simulink model "flug2d2"  (Simulink 7.0)
settings: Solver=ode45  StartTime=0.0  StopTime=700  RelTol=1e-3
libraries: kalmanlib x2, simulink x2
settings Model: Creator=peter  LastModifiedBy=peter  ExtModeAutoUpdateStatusClock=off

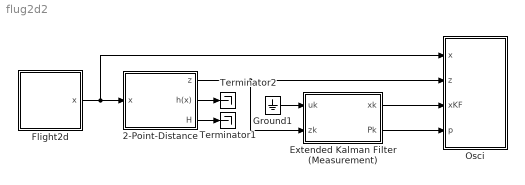
== system flug2d2 ==
  2-Point-Distance : Subsystem  mask(twoPointDistance){P1=[1000;4000], P2=[3000;0], R=diag([1 1 0.003 0.003]), dt=1, seed=[1 2 3 4]'}
      mask prompts: P1 "1. Bezugspunkt"; P2 "2. Bezugspunkt"; R "variance of  measurement noise R"; dt "sample time"; seed "initial seed"
      mask help:
      | Measurement z = h(x) given by the distance to two fixed points P1, P2.
      | Assumes input vector of the form (x, y, vx, vy, ax, ay).
      |
      | returns h(x) and the Jacobi Matrix H
  Extended Kalman Filter (Measurement) : Subsystem  mask(Kalman Filter){A=kron([1, 1, 0.5; 0, 1, 1;  0, 0, 1], [1, 0; 0, 1]), B=0, Q=kron([0.050,0.125,0.167; 0.125,0.333,0.500; 0.167,0.500,1.000],[1, 0; 0, 1])*0.001, R=[1 0 0 0; 0 1 0 0; 0 0 0.003 0; 0 0 0 0.003], x0=[50 4001 0 0 0 0]', P0=diag([1 1 1 1 1 1])*1e-2}
      mask prompts: A "Übertragungsmatrix A"; B "Kontrollmatrix B"; Q "Varianz der x-Störung Q"; R "Varianz der y-Störung R"; x0 "geschätzter Anfangsvektor x0"; P0 "geschätzte x-Anfangsvarianz P"
      mask Display:
      | disp('EKF (M)')
      | port_label('input', 1, 'u')
      | port_label('input', 2, 'z')
      | port_label('output', 1, 'x')
      | port_label('output', 2, 'P')
  Flight2d : Subsystem  mask(Flight2D){xS=[50;4000], xL=[4500;50], tS=50, tL=70, v0=10, q=0.001, dt=1, seed=17, s=0, tF=0, e=0}
      mask prompts: xS "start point"; xL "landing point"; tS "duration of start"; tL "duration of landing"; v0 "cruise velocity"; q "variance of acceleration"; dt "sample time"; seed "initial seed"; s "total distance"; tF "cruise time"; e "cruise vector"
      mask init:
      | s = norm(xL - xS);
      | tF = (s - v0/2*(tS + tL))/v0;
      | e = (xL - xS)/s;
      mask Display:
      | plot([0.1 0.8], [0.1 0.9])
      | patch(0.1 + 0.05*cos(0:0.2:2*pi), 0.1 + 0.05*sin(0:0.2:2*pi), [1 0 0])
      | patch(0.8 + 0.05*cos(0:0.2:2*pi), 0.9 + 0.05*sin(0:0.2:2*pi), [1 0 0])
      | port_label('output', 1, 'x')
  Ground1 : Ground
  Osci : Subsystem
      settings: OpenFcn=open_system(find_system(gcbh, 'Name', 'Scope'), 'force')
  Terminator1 : Terminator
  Terminator2 : Terminator
  wires:
  Flight2d/1(x) -> 2-Point-Distance/1(x), Osci/1(x)
  Ground1/1 -> Extended Kalman Filter (Measurement)/1(uk)
  2-Point-Distance/1(z) -> Extended Kalman Filter (Measurement)/2(zk), Osci/2(z)
  Extended Kalman Filter (Measurement)/1(xk) -> Osci/3(xKF)
  Extended Kalman Filter (Measurement)/2(Pk) -> Osci/4(p)
  2-Point-Distance/2(h(x)) -> Terminator2/1
  2-Point-Distance/3(H) -> Terminator1/1

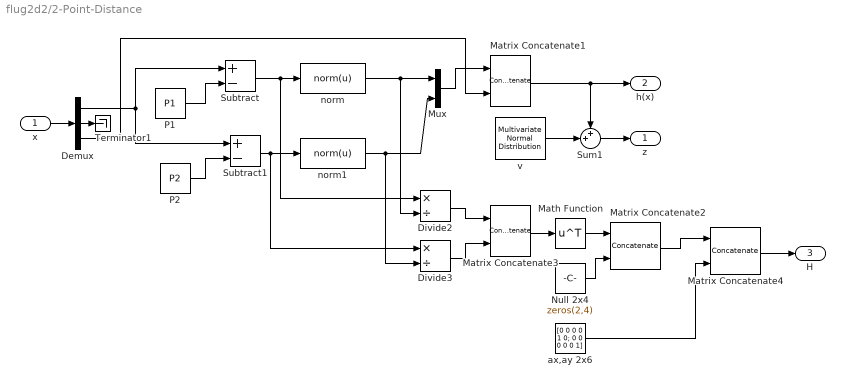
== system flug2d2/2-Point-Distance ==
  x : Inport  OutDataType=sfix(16)  OutScaling=2^0
  Demux : Demux  Outputs=3
  Divide2 : Product  Inputs=*/  OutDataType=sfix(16)  OutScaling=2^-10
  Divide3 : Product  Inputs=*/  OutDataType=sfix(16)  OutScaling=2^-10
  Math Function : Math  Operator=transpose  OutDataType=sfix(16)  OutScaling=2^0  SaturateOnIntegerOverflow=on
  Matrix Concatenate1 : Concatenate  Mode=Multidimensional array
  Matrix Concatenate2 : Concatenate  Mode=Multidimensional array  ConcatenateDimension=2
  Matrix Concatenate3 : Concatenate  Mode=Multidimensional array  ConcatenateDimension=2
  Matrix Concatenate4 : Concatenate  Mode=Multidimensional array
  Mux : Mux  Inputs=2
  Null 2x4 : Constant  Value=zeros(2,4)  VectorParams1D=off  OutDataType=sfix(16)  OutScaling=2^0
  P1 : Constant  Value=P1  VectorParams1D=off  OutDataType=sfix(16)  OutScaling=2^0
  P2 : Constant  Value=P2  VectorParams1D=off  OutDataType=sfix(16)  OutScaling=2^0
  Subtract : Sum  Inputs=+-  OutDataType=sfix(16)  OutScaling=2^-10
  Subtract1 : Sum  Inputs=+-  OutDataType=sfix(16)  OutScaling=2^-10
  Sum1 : Sum  Inputs=++|  OutDataType=sfix(16)  OutScaling=2^0
  Terminator1 : Terminator
  ax,ay 2x6 : Constant  Value=[0 0 0 0 1 0; 0 0 0 0 0 1]  VectorParams1D=off  OutDataType=sfix(16)  OutScaling=2^0
  norm : MATLABFcn  MATLABFcn=norm(u)  OutputDimensions=1
  norm1 : MATLABFcn  MATLABFcn=norm(u)  OutputDimensions=1
  v : kalmanlib/auxiliary/Multivariate Normal  Distribution  SystemSampleTime=-1  m=0  P=R  seed=seed  tS=dt  C=0
  z : Outport  OutDataType=sfix(16)  OutScaling=2^0
  h(x) : Outport  Port=2  OutDataType=sfix(16)  OutScaling=2^0
  H : Outport  Port=3  OutDataType=sfix(16)  OutScaling=2^0
  wires:
  Matrix Concatenate3/1 -> Math Function/1
  Null 2x4/1 -> Matrix Concatenate2/2
  Divide3/1 -> Matrix Concatenate3/2
  Divide2/1 -> Matrix Concatenate3/1
  norm1/1 -> Divide3/2, Mux/2
  norm/1 -> Divide2/2, Mux/1
  Subtract1/1 -> Divide3/1, norm1/1
  Subtract/1 -> Divide2/1, norm/1
  P2/1 -> Subtract1/2
  P1/1 -> Subtract/2
  Demux/1 -> Subtract/1, Subtract1/1
  x/1 -> Demux/1
  Sum1/1 -> z/1
  v/1 -> Sum1/2
  Math Function/1 -> Matrix Concatenate2/1
  Demux/2 -> Terminator1/1
  Mux/1 -> Matrix Concatenate1/1
  Demux/3 -> Matrix Concatenate1/2
  Matrix Concatenate1/1 -> Sum1/1, h(x)/1
  Matrix Concatenate2/1 -> Matrix Concatenate4/1
  ax,ay 2x6/1 -> Matrix Concatenate4/2
  Matrix Concatenate4/1 -> H/1

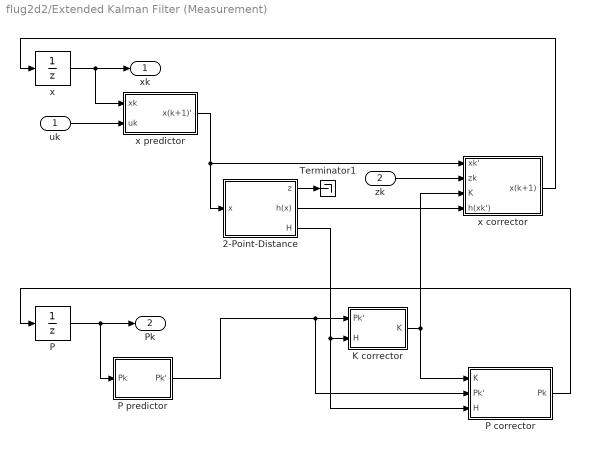
== system flug2d2/Extended Kalman Filter (Measurement) ==
  uk : Inport  OutDataType=sfix(16)  OutScaling=2^0
  zk : Inport  Port=2  OutDataType=sfix(16)  OutScaling=2^0
  2-Point-Distance : Subsystem  mask(twoPointDistance){P1=[1000;4000], P2=[3000;0], R=R, dt=1, seed=[1 2 3 4]'}
      mask prompts: P1 "1. Bezugspunkt"; P2 "2. Bezugspunkt"; R "variance of  measurement noise R"; dt "sample time"; seed "initial seed"
      mask help:
      | Measurement z = h(x) given by the distance to two fixed points P1, P2.
      | Assumes input vector of the form (x, y, vx, vy, ax, ay).
      |
      | returns h(x) and the Jacobi Matrix H
  K corrector : Subsystem
  P : UnitDelay  X0=P0  SampleTime=-1
  P corrector : Subsystem
  P predictor : Subsystem
  Terminator1 : Terminator
  x : UnitDelay  X0=x0  SampleTime=-1
  x corrector : Subsystem
  x predictor : Subsystem
  xk : Outport  OutDataType=sfix(16)  OutScaling=2^0
  Pk : Outport  Port=2  OutDataType=sfix(16)  OutScaling=2^0
  wires:
  2-Point-Distance/3(H) -> P corrector/3(H), K corrector/2(H)
  2-Point-Distance/2(h(x)) -> x corrector/4(h(xk'))
  x corrector/1(x(k+1)) -> x/1
  x/1 -> x predictor/1(xk), xk/1
  P corrector/1(Pk) -> P/1
  K corrector/1(K) -> P corrector/1(K), x corrector/3(K)
  P predictor/1(Pk') -> K corrector/1(Pk'), P corrector/2(Pk')
  P/1 -> Pk/1, P predictor/1(Pk)
  x predictor/1(x(k+1)') -> x corrector/1(xk'), 2-Point-Distance/1(x)
  zk/1 -> x corrector/2(zk)
  uk/1 -> x predictor/2(uk)
  2-Point-Distance/1(z) -> Terminator1/1

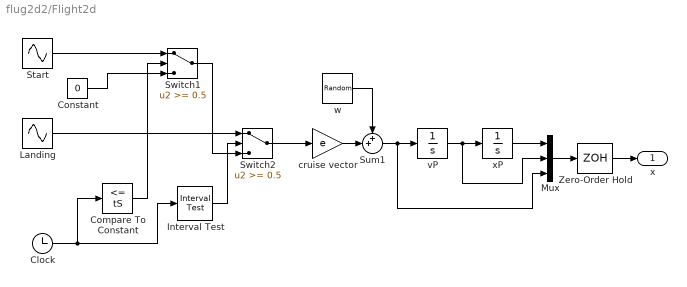
== system flug2d2/Flight2d ==
  Clock : Clock
      settings: Decimation=10
  Compare To Constant : simulink/Logic and Bit Operations/Compare To Constant  SystemSampleTime=-1  relop=<=  const=tS  LogicOutDataTypeMode=boolean  ZeroCross=off
  Constant : Constant  Value=0  OutDataType=sfix(16)  OutScaling=2^0
  Interval Test : simulink/Logic and Bit Operations/Interval Test  SystemSampleTime=-1  IntervalClosedRight=on  uplimit=tS+tF+tL  IntervalClosedLeft=on  lowlimit=tS+tF  LogicOutDataTypeMode=boolean
  Landing : Sin  Amplitude=-v0*pi/(2*tL)  Frequency=pi/tL  Phase=-pi*(tS+tF)/tL  SampleTime=0
  Mux : Mux  Inputs=3
  Start : Sin  Amplitude=v0*pi/(2*tS)  Frequency=pi/tS  SampleTime=0
  Sum1 : Sum  Inputs=++|  OutDataType=sfix(16)  OutScaling=2^0
  Switch1 : Switch  Threshold=0.5
  Switch2 : Switch  Threshold=0.5
  Zero-Order Hold : ZeroOrderHold  SampleTime=dt
  cruise vector : Gain  Gain=e  ParameterDataType=sfix(16)  ParameterScaling=2^0  OutDataType=sfix(16)  OutScaling=2^0
  vP : Integrator  InitialCondition=[0;0]
  w : RandomNumber  Variance=q  Seed=[seed; seed+1]  SampleTime=dt  VectorParams1D=off
  xP : Integrator  InitialCondition=xS
  x : Outport  OutDataType=sfix(16)  OutScaling=2^0
  wires:
  Start/1 -> Switch1/1
  Constant/1 -> Switch1/3
  Compare To Constant/1 -> Switch1/2
  Clock/1 -> Compare To Constant/1, Interval Test/1
  Interval Test/1 -> Switch2/2
  Switch1/1 -> Switch2/3
  Landing/1 -> Switch2/1
  vP/1 -> xP/1, Mux/2
  xP/1 -> Mux/1
  Mux/1 -> Zero-Order Hold/1
  Switch2/1 -> cruise vector/1
  Sum1/1 -> vP/1, Mux/3
  w/1 -> Sum1/1
  Zero-Order Hold/1 -> x/1
  cruise vector/1 -> Sum1/2

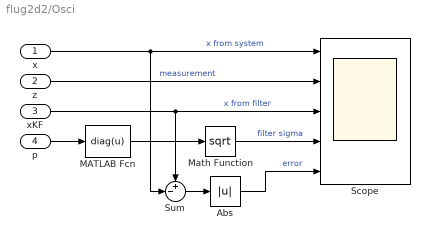
== system flug2d2/Osci ==
  x : Inport  OutDataType=sfix(16)  OutScaling=2^0
  z : Inport  Port=2  OutDataType=sfix(16)  OutScaling=2^0
  xKF : Inport  Port=3  OutDataType=sfix(16)  OutScaling=2^0
  p : Inport  Port=4  OutDataType=sfix(16)  OutScaling=2^0
  Abs : Abs
  MATLAB Fcn : MATLABFcn  MATLABFcn=diag(u)
  Math Function : Math  Operator=sqrt  OutDataType=sfix(16)  OutScaling=2^0  SaturateOnIntegerOverflow=on
  Scope : Scope  NumInputPorts=5
      settings: TimeRange=700  YMin=-1000~-1000~-1000~0~0  YMax=5000~6000~5000~10~30
  Sum : Sum  Inputs=+-|  OutDataType=sfix(16)  OutScaling=2^0
  wires:
  p/1 -> MATLAB Fcn/1
  xKF/1 -> Sum/1, Scope/3  "x from filter"
  z/1 -> Scope/2  "measurement"
  x/1 -> Sum/2, Scope/1  "x from system"
  Abs/1 -> Scope/5  "error"
  Sum/1 -> Abs/1
  Math Function/1 -> Scope/4  "filter sigma"
  MATLAB Fcn/1 -> Math Function/1

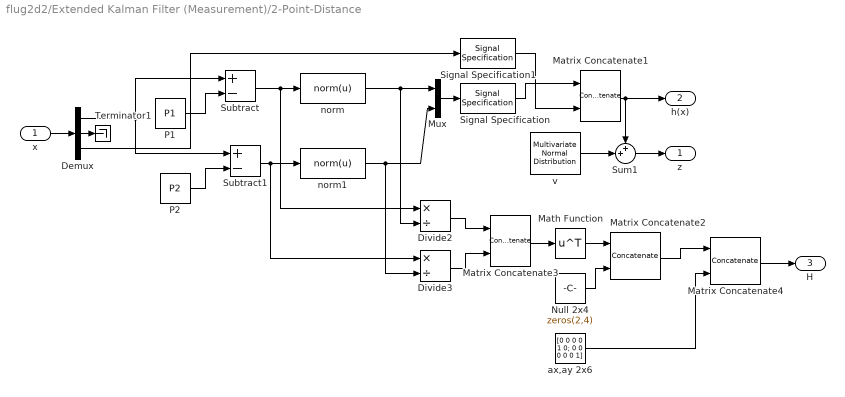
== system flug2d2/Extended Kalman Filter (Measurement)/2-Point-Distance ==
  x : Inport  OutDataType=sfix(16)  OutScaling=2^0
  Demux : Demux  Outputs=3
  Divide2 : Product  Inputs=*/  OutDataType=sfix(16)  OutScaling=2^-10
  Divide3 : Product  Inputs=*/  OutDataType=sfix(16)  OutScaling=2^-10
  Math Function : Math  Operator=transpose  OutDataType=sfix(16)  OutScaling=2^0  SaturateOnIntegerOverflow=on
  Matrix Concatenate1 : Concatenate  Mode=Multidimensional array
  Matrix Concatenate2 : Concatenate  Mode=Multidimensional array  ConcatenateDimension=2
  Matrix Concatenate3 : Concatenate  Mode=Multidimensional array  ConcatenateDimension=2
  Matrix Concatenate4 : Concatenate  Mode=Multidimensional array
  Mux : Mux  Inputs=2
  Null 2x4 : Constant  Value=zeros(2,4)  VectorParams1D=off  OutDataType=sfix(16)  OutScaling=2^0
  P1 : Constant  Value=P1  VectorParams1D=off  OutDataType=sfix(16)  OutScaling=2^0
  P2 : Constant  Value=P2  VectorParams1D=off  OutDataType=sfix(16)  OutScaling=2^0
  Signal Specification : SignalSpecification  Dimensions=[2 1]  OutDataType=sfix(16)  OutScaling=2^0
  Signal Specification1 : SignalSpecification  Dimensions=[2 1]  OutDataType=sfix(16)  OutScaling=2^0
  Subtract : Sum  Inputs=+-  OutDataType=sfix(16)  OutScaling=2^-10
  Subtract1 : Sum  Inputs=+-  OutDataType=sfix(16)  OutScaling=2^-10
  Sum1 : Sum  Inputs=++|  OutDataType=sfix(16)  OutScaling=2^0
  Terminator1 : Terminator
  ax,ay 2x6 : Constant  Value=[0 0 0 0 1 0; 0 0 0 0 0 1]  VectorParams1D=off  OutDataType=sfix(16)  OutScaling=2^0
  norm : MATLABFcn  MATLABFcn=norm(u)  OutputDimensions=1
  norm1 : MATLABFcn  MATLABFcn=norm(u)  OutputDimensions=1
  v : kalmanlib/auxiliary/Multivariate Normal  Distribution  SystemSampleTime=-1  m=0  P=R  seed=seed  tS=dt  C=0
  z : Outport  OutDataType=sfix(16)  OutScaling=2^0
  h(x) : Outport  Port=2  OutDataType=sfix(16)  OutScaling=2^0
  H : Outport  Port=3  OutDataType=sfix(16)  OutScaling=2^0
  wires:
  Signal Specification1/1 -> Matrix Concatenate1/2
  Signal Specification/1 -> Matrix Concatenate1/1
  Matrix Concatenate4/1 -> H/1
  ax,ay 2x6/1 -> Matrix Concatenate4/2
  Matrix Concatenate2/1 -> Matrix Concatenate4/1
  Matrix Concatenate1/1 -> h(x)/1, Sum1/1
  Demux/3 -> Signal Specification1/1
  Mux/1 -> Signal Specification/1
  Demux/2 -> Terminator1/1
  Math Function/1 -> Matrix Concatenate2/1
  v/1 -> Sum1/2
  Sum1/1 -> z/1
  x/1 -> Demux/1
  Demux/1 -> Subtract1/1, Subtract/1
  P1/1 -> Subtract/2
  P2/1 -> Subtract1/2
  Subtract/1 -> norm/1, Divide2/1
  Subtract1/1 -> norm1/1, Divide3/1
  norm/1 -> Mux/1, Divide2/2
  norm1/1 -> Mux/2, Divide3/2
  Divide2/1 -> Matrix Concatenate3/1
  Divide3/1 -> Matrix Concatenate3/2
  Null 2x4/1 -> Matrix Concatenate2/2
  Matrix Concatenate3/1 -> Math Function/1

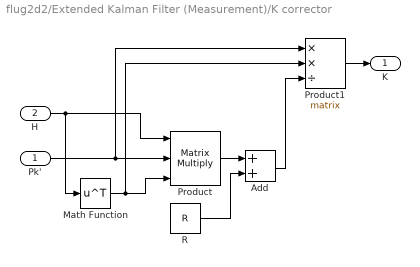
== system flug2d2/Extended Kalman Filter (Measurement)/K corrector ==
  Pk' : Inport  OutDataType=sfix(16)  OutScaling=2^0
  H : Inport  Port=2  OutDataType=sfix(16)  OutScaling=2^0
  Add : Sum  OutDataType=sfix(16)  OutScaling=2^-10
  Math Function : Math  Operator=transpose  OutDataType=sfix(16)  OutScaling=2^0  SaturateOnIntegerOverflow=on
  Product : Product  Inputs=3  Multiplication=Matrix(*)  OutDataType=sfix(16)  OutScaling=2^0  RndMeth=Zero
  Product1 : Product  Inputs=**/  Multiplication=Matrix(*)  OutDataType=sfix(16)  OutScaling=2^0  RndMeth=Zero
  R : Constant  Value=R  OutDataType=sfix(16)  OutScaling=2^0
  K : Outport  OutDataType=sfix(16)  OutScaling=2^0
  wires:
  Add/1 -> Product1/3
  Product1/1 -> K/1
  H/1 -> Math Function/1, Product/1
  Pk'/1 -> Product1/1, Product/2
  Math Function/1 -> Product1/2, Product/3
  Product/1 -> Add/1
  R/1 -> Add/2

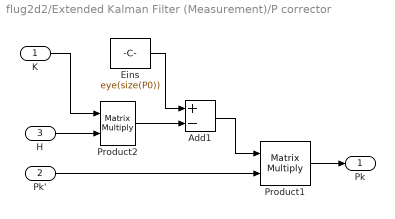
== system flug2d2/Extended Kalman Filter (Measurement)/P corrector ==
  K : Inport  OutDataType=sfix(16)  OutScaling=2^0
  Pk' : Inport  Port=2  OutDataType=sfix(16)  OutScaling=2^0
  H : Inport  Port=3  OutDataType=sfix(16)  OutScaling=2^0
  Add1 : Sum  Inputs=+-  OutDataType=sfix(16)  OutScaling=2^-10
  Eins : Constant  Value=eye(size(P0))  VectorParams1D=off  OutDataType=sfix(16)  OutScaling=2^0
  Product1 : Product  Multiplication=Matrix(*)  OutDataType=sfix(16)  OutScaling=2^0  RndMeth=Zero
  Product2 : Product  Multiplication=Matrix(*)  OutDataType=sfix(16)  OutScaling=2^0  RndMeth=Zero
  Pk : Outport  OutDataType=sfix(16)  OutScaling=2^0
  wires:
  H/1 -> Product2/2
  K/1 -> Product2/1
  Add1/1 -> Product1/1
  Eins/1 -> Add1/1
  Product2/1 -> Add1/2
  Pk'/1 -> Product1/2
  Product1/1 -> Pk/1

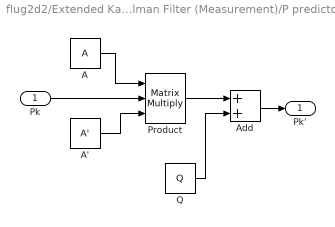
== system flug2d2/Extended Kalman Filter (Measurement)/P predictor ==
  Pk : Inport  OutDataType=sfix(16)  OutScaling=2^0
  A : Constant  Value=A  OutDataType=sfix(16)  OutScaling=2^0
  A' : Constant  Value=A'  OutDataType=sfix(16)  OutScaling=2^0
  Add : Sum  OutDataType=sfix(16)  OutScaling=2^-10
  Product : Product  Inputs=3  Multiplication=Matrix(*)  OutDataType=sfix(16)  OutScaling=2^0  RndMeth=Zero
  Q : Constant  Value=Q  VectorParams1D=off  OutDataType=sfix(16)  OutScaling=2^0
  Pk' : Outport  OutDataType=sfix(16)  OutScaling=2^0
  wires:
  Add/1 -> Pk'/1
  Q/1 -> Add/2
  Product/1 -> Add/1
  A'/1 -> Product/3
  Pk/1 -> Product/2
  A/1 -> Product/1

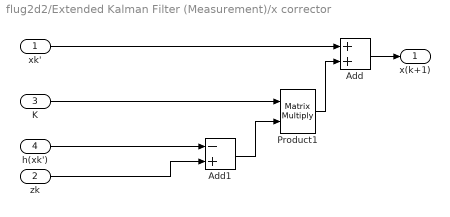
== system flug2d2/Extended Kalman Filter (Measurement)/x corrector ==
  xk' : Inport  OutDataType=sfix(16)  OutScaling=2^0
  zk : Inport  Port=2  OutDataType=sfix(16)  OutScaling=2^0
  K : Inport  Port=3  OutDataType=sfix(16)  OutScaling=2^0
  h(xk') : Inport  Port=4  OutDataType=sfix(16)  OutScaling=2^0
  Add : Sum  OutDataType=sfix(16)  OutScaling=2^-10
  Add1 : Sum  Inputs=-+  OutDataType=sfix(16)  OutScaling=2^-10
  Product1 : Product  Multiplication=Matrix(*)  OutDataType=sfix(16)  OutScaling=2^0  RndMeth=Zero
  x(k+1) : Outport  OutDataType=sfix(16)  OutScaling=2^0
  wires:
  h(xk')/1 -> Add1/1
  Add1/1 -> Product1/2
  zk/1 -> Add1/2
  K/1 -> Product1/1
  Product1/1 -> Add/2
  xk'/1 -> Add/1
  Add/1 -> x(k+1)/1

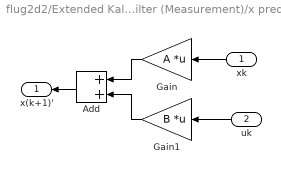
== system flug2d2/Extended Kalman Filter (Measurement)/x predictor ==
  xk : Inport  Orientation=left  OutDataType=sfix(16)  OutScaling=2^0
  uk : Inport  Orientation=left  Port=2  OutDataType=sfix(16)  OutScaling=2^0
  Add : Sum  Orientation=left  OutDataType=sfix(16)  OutScaling=2^-10
  Gain : Gain  Orientation=left  Gain=A  Multiplication=Matrix(K*u)  ParameterDataType=sfix(16)  ParameterScaling=2^0  OutDataType=sfix(16)  OutScaling=2^0
  Gain1 : Gain  Orientation=left  Gain=B  Multiplication=Matrix(K*u)  ParameterDataType=sfix(16)  ParameterScaling=2^0  OutDataType=sfix(16)  OutScaling=2^0
  x(k+1)' : Outport  Orientation=left  OutDataType=sfix(16)  OutScaling=2^0
  wires:
  xk/1 -> Gain/1
  uk/1 -> Gain1/1
  Gain/1 -> Add/1
  Gain1/1 -> Add/2
  Add/1 -> x(k+1)'/1
